simulink model "SimulationSorting"  (R2024b)
settings: Solver=VariableStepAuto  StartTime=0.0  StopTime=Inf  RelTol=1e-3
PreLoadFcn:
  | addpath(genpath(pwd))
  | load("model_data.mat");
undefined symbols (not defined in the file): gray, q_grip1, Sim3dSensor
libraries: sim3dlib x5, robotcorelib x1, robotmaniplib x1, sim3dcameralib x1, robotsim3dlib x1
settings Model: Creator=gbhosale  LastModifiedBy=10177

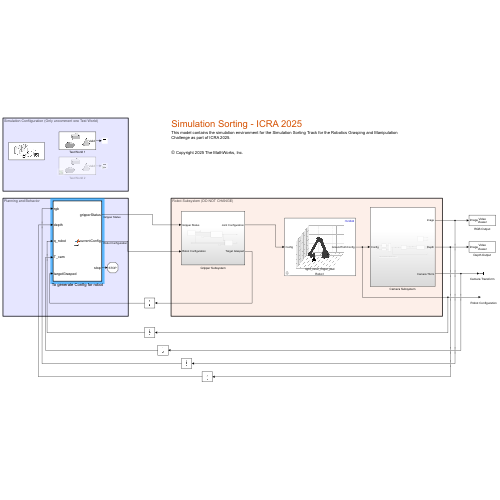
[thumbnail: Simulink's stored preview of the top-level diagram]
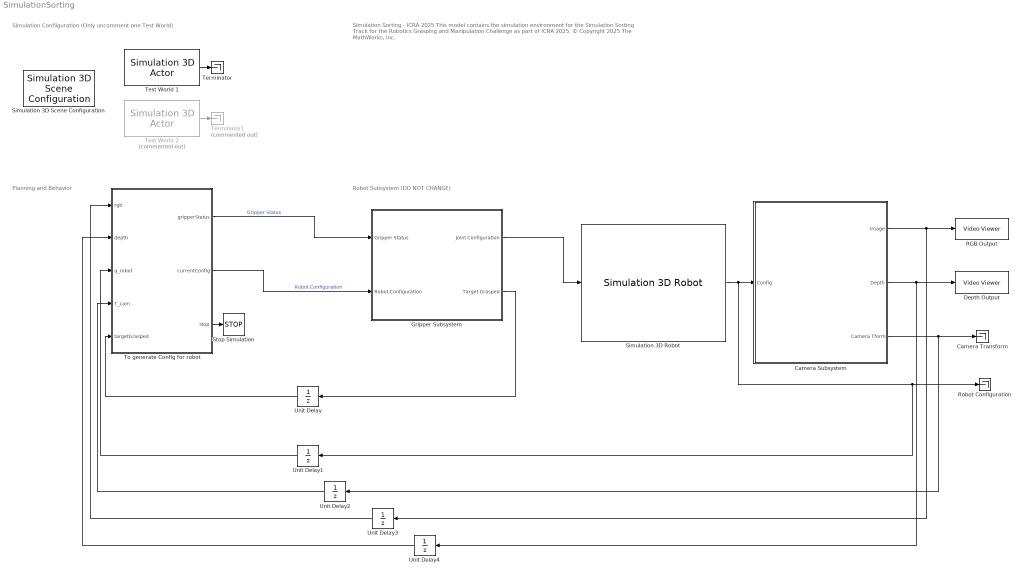
== system SimulationSorting ==
  note: Robot Subsystem (DO NOT CHANGE)
  note: Planning and Behavior
  note: Simulation Confiiguration (Only uncomment one Test World)
  note: Simulation Sorting - ICRA 2025
      | This model contains the simulation environment for the Simulation Sorting Track for the Robotics Grasping and Manipulation Challenge as part of ICRA 2025.
      |
      | © Copyright 2025 The MathWorks, Inc.
  Camera Subsystem : Subsystem
  Camera Transform : Terminator
  Depth Output : VideoViewer  colormapValue=gray(256)  FigPos=[886.5 747 400.5 311]
  Gripper Subsystem : Subsystem
  RGB Output : VideoViewer  colormapValue=gray(256)  FigPos=[892.5 410 400 305]
  Robot Configuration : Terminator
  Simulation 3D Robot : robotsim3dlib/Simulation 3D Robot  actorInputType=RigidBodyTree Object  RigidBodyTree=rt.robot  ActorName=Robo1  existActorChekBox=on  initialTrans=[nan nan nan]  initialRot=[ 0 0 0]  initialConfig=[-0.2618 -2.1991 1.9722 -1.3963 -1.5882 1.3265 0 0 0 0 0 0]  EndEffector=right_inner_finger_pad  eeOffsetInpChekBox=off  eeTargetTrans=[ 0 0 0.08 ]  eeTargetRot=[ 0 0 0 ]  enableRegionGraspChekBox=off  regionGraspInpChekBox=on  eeTargTransDiff=[ 0.001 0.001 2 ]  eeTargRotDiff=[ nan nan nan ]  inpConfEnbVal=on  inpGraspEnbVal=off  inpTransEnbVal=off  outConfEnbVal=on  outGraspEnbVal=off  outTransEnbVal=off  SampleTime=0.01  ActorType=SimulinkVehicle  ID=C  aMode=6  ActorTag=Robo1  Mesh=RigidBodyTree
  Simulation 3D Scene Configuration : sim3dlib/Simulation 3D Scene Configuration  Priority=0  ProjectFormat=Unreal Executable  SceneDesc=Empty scene  ProjectName=SimSort_Env_Executable\VehicleSimulation.exe  ScenePath=/Game/Maps/EmptyScene  EnableOpenDRIVE=off  vehTagList={'Custom';'Robo1';'Scene Origin';'Sim3dActor2';'Sim3dActor3';'SimSortWorld';'cameraPlaceHolder'}  vehTag=Scene Origin  FreeCameraInitialTranslation=[0, 0, 0]  FreeCameraDefaultInitialTranslation=[-6, 0, 2]  FreeCameraInitialRotation=[0, 0, 0]  FreeCameraDefaultInitialRotation=[0, -15, 0]  OpVisEn=off  Ts=0.01  EnableWindow=on  EnableRemoteAccess=off  EnableWeather=off  SunAzimuth=90  SunAltitude=40.0  EnableGeospatialSun=off  Latitude=0  Longitude=0  Date=2023-01-01  Time=10:30:00  GeoTimeZone=-5.0  SunDaylightSaving=off  wind=1  clouds=10  EnableVolumetricClouds=off  CloudCoverage=0  CloudAltitude=6  fog=0  rain=0  RaindropsEffect=off  SnowDensity=0  EnableGeospatial=off  UseTrueOrigin=off  OriginHeight=200  OriginLatitude=40.744652  OriginLongitude=-73.988864  MapStyle=Aerial  AdditionalAssetIDs=[]  UseAdvancedSunSky=off  SolarTime=11  TimeZone=-5  Day=21  Month=9  Year=2022  UseDaylightSavingTime=on  DSTStartDay=10  DSTStartMonth=3  DSTEndDay=3  DSTEndMonth=11  DSTSwitchHour=2  sensorTag=MainCamera1  sensorId=1  sensorName=MainCamera1  mountLoc=Origin  offsetFlag=off  tmountOffset=[0, 0, 0]  rmountOffset=[0, 0, 0]  HorizontalResolution=1280  VerticalResolution=720  HorizontalFOV=60  mountPoint=[0 0 0]  mountOrientation=[0 0 0]  aMode=6  ID=1  GeoTrigger=Inactive
      settings: LibrarySourceBlock=robotsim3dlib/Simulation 3D Scene Configuration
  Stop Simulation : Stop
  Terminator : Terminator
  Terminator1 : Terminator  Commented=on
  Test World 1 : sim3dlib/Simulation 3D Actor  Priority=1  ActorName=SimSortWorld  ParentName=Scene Origin  Operation=Create at setup  InitScriptText=|  SampleTime=-1  Translation=[0 0 0]  Rotation=[0 0 0]  Scale=[1 1 1]  aMode=5  ActorTag=SimSortWorld  ActorType=Sim3dActor  ID=C
      | % Reserved keywords:
      | % - Actor : handle to this actor object
      | % - World : handle to the world object
      | 
      | % Examples:
      | 
      | % Create a primitive geometry (optional)
      | % createShape(Actor, 'box', [1 1 1]);
      | 
      | % Initialize values (optional)
      | % Actor.Physics = true;
      | % Actor.Color = [1 0 0];
      | 
      | Actor.load('simSortWorld1.mat')
  Test World 2 : sim3dlib/Simulation 3D Actor  Priority=1  Commented=on  ActorName=Sim3dActor3  ParentName=Scene Origin  Operation=Create at setup  InitScriptText=|  SampleTime=-1  Translation=[0 0 0]  Rotation=[0 0 0]  Scale=[1 1 1]  aMode=5  ActorTag=Sim3dActor3  ActorType=Sim3dActor  ID=3
      | % Reserved keywords:
      | % - Actor : handle to this actor object
      | % - World : handle to the world object
      | 
      | % Examples:
      | 
      | % Create a primitive geometry (optional)
      | % createShape(Actor, 'box', [1 1 1]);
      | 
      | % Initialize values (optional)
      | % Actor.Physics = true;
      | % Actor.Color = [1 0 0];
      | 
      | Actor.load('simSortWorld2.mat')
  To generate Config for robot : MATLAB Function  TreatAsAtomicUnit=on
  Unit Delay{,1..4} (5 alike) : UnitDelay  SampleTime=-1  HasFrameUpgradeWarning=on
  wires:
  To generate Config for robot/3(stop) -> Stop Simulation/1
  Simulation 3D Robot/1 -> Camera Subsystem/1(Config), Unit Delay1/1, Robot Configuration/1
  Test World 1/1 -> Terminator/1
  Test World 2/1 -> Terminator1/1
  To generate Config for robot/1(gripperStatus) -> Gripper Subsystem/1(Gripper Status)  "Gripper Status"
  To generate Config for robot/2(currentConfig) -> Gripper Subsystem/2(Robot Configuration)  "Robot Configuration"
  Gripper Subsystem/1(Joint Configuration) -> Simulation 3D Robot/1
  Gripper Subsystem/2(Target Grasped) -> Unit Delay/1
  Unit Delay/1 -> To generate Config for robot/5(targetGrasped)
  Camera Subsystem/1(Image) -> Unit Delay3/1, RGB Output/1
  Camera Subsystem/2(Depth) -> Unit Delay4/1, Depth Output/1
  Camera Subsystem/3(Camera Tform) -> Unit Delay2/1, Camera Transform/1
  Unit Delay1/1 -> To generate Config for robot/3(q_robot)
  Unit Delay2/1 -> To generate Config for robot/4(T_cam)
  Unit Delay4/1 -> To generate Config for robot/2(depth)
  Unit Delay3/1 -> To generate Config for robot/1(rgb)

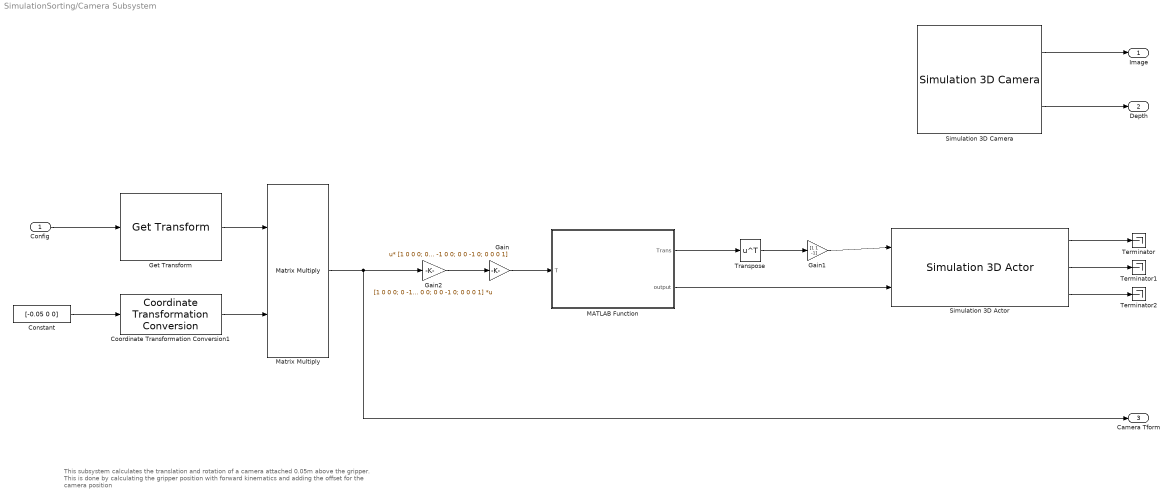
== system SimulationSorting/Camera Subsystem ==
  note: This subsystem calculates the translation and rotation of a camera attached 0.05m above the gripper. This is done by calculating the gripper position with forward kinematics and adding the offset for the camera position
  Config : Inport
  Constant : Constant  Value=[-0.05 0 0]
  Coordinate Transformation Conversion1 : robotcorelib/Coordinate Transformation Conversion  InputRepresentation=Translation Vector  InputEulerSequence=ZYX  ShowTrVecInputPort=on  OutputRepresentation=Homogeneous Transformation  OutputEulerSequence=ZYX  ShowTrVecOutputPort=on  SimulateUsing=Interpreted execution
  Gain : Gain  Gain=[1 0 0 0; 0 -1 0 0; 0 0 -1 0; 0 0 0 1]  Multiplication=Matrix(u*K)
  Gain1 : Gain  Gain=[1 1 -1]
  Gain2 : Gain  Gain=[1 0 0 0; 0 -1 0 0; 0 0 -1 0; 0 0 0 1]  Multiplication=Matrix(K*u)
  Get Transform : robotmaniplib/Get Transform  RigidBodyTree=rt.robot  SourceBody=robotiq_arg2f_base_link  TargetBody=base_link  SimulateUsing=Interpreted execution
  MATLAB Function : MATLAB Function  TreatAsAtomicUnit=on
  Matrix Multiply : Product  Multiplication=Matrix(*)
  Simulation 3D Actor : sim3dlib/Simulation 3D Actor  Priority=1  ActorName=cameraPlaceHolder  ParentName=Robo1  Operation=Create at setup  InitScriptText=|  SampleTime=-1  Translation=[0.05 0 0]  Rotation=[0 0 0]  Scale=[1 1 1]  InputsText=cameraPlaceHolder.Translation cameraPlaceHolder.Rotation  OutputsText=cameraPlaceHolder.Translation cameraPlaceHolder.Rotation  aMode=5  ActorTag=cameraPlaceHolder  ActorType=Sim3dActor  ID=C
      | Actor.createShape('box', [0.02 0.04 0.06]);
      | Actor.Mobility=sim3d.utils.MobilityTypes.Movable;
      | Actor.Color=[1 0 0];
      | Actor.Translation=[0.05, 0, 0];
      | Actor.Rotation = [0, 0, 0];
      | Actor.ConstantAttributes=false;
      | Actor.Mass = 1;
      | Actor.Transparency = 0;
      | Actor.Shininess = 0;
  Simulation 3D Camera : sim3dcameralib/Simulation 3D Camera  Priority=1  sensorTag=Sim3dSensor�  sensorId=3  sensorName=Sim3dSensor�  vehTagList={'Robo1';'Scene Origin';'Sim3dActor2';'Sim3dActor3';'SimSortWorld';'cameraPlaceHolder'}  vehTag=cameraPlaceHolder  mountLoc=Origin  offsetFlag=on  tmountOffset=[0 0 0]  extTmount=off  rmountOffset=[0, -90, 0]  extRmount=off  FocalLength=[1109, 1109]  OpticalCenter=[640, 360]  ImageSize=[720, 1280]  RadialDistortion=[0, 0]  TangentialDistortion=[0, 0]  SensorSkew=0  DepthOutportEnabled=on  SemanticOutportEnabled=off  TransformOutportEnabled=off  SampleTime=0.01  mountPoint=[0 0 0]  mountOrientation=[0 90 0]  aMode=5  ID=3
      settings: LibrarySourceBlock=Simulation 3D Camera
  Terminator : Terminator
  Terminator1 : Terminator
  Terminator2 : Terminator
  Transpose : Math  Operator=transpose
  Image : Outport
  Depth : Outport  Port=2
  Camera Tform : Outport  Port=3
  wires:
  Config/1 -> Get Transform/1
  Coordinate Transformation Conversion1/1 -> Matrix Multiply/2
  Get Transform/1 -> Matrix Multiply/1
  Constant/1 -> Coordinate Transformation Conversion1/1
  Matrix Multiply/1 -> Camera Tform/1, Gain2/1
  Simulation 3D Camera/1 -> Image/1
  Simulation 3D Camera/2 -> Depth/1
  Gain2/1 -> Gain/1
  Gain/1 -> MATLAB Function/1(T)
  MATLAB Function/1(Trans) -> Transpose/1
  Transpose/1 -> Gain1/1
  Gain1/1 -> Simulation 3D Actor/1
  MATLAB Function/2(output) -> Simulation 3D Actor/2
  Simulation 3D Actor/3 -> Terminator2/1
  Simulation 3D Actor/2 -> Terminator1/1
  Simulation 3D Actor/1 -> Terminator/1

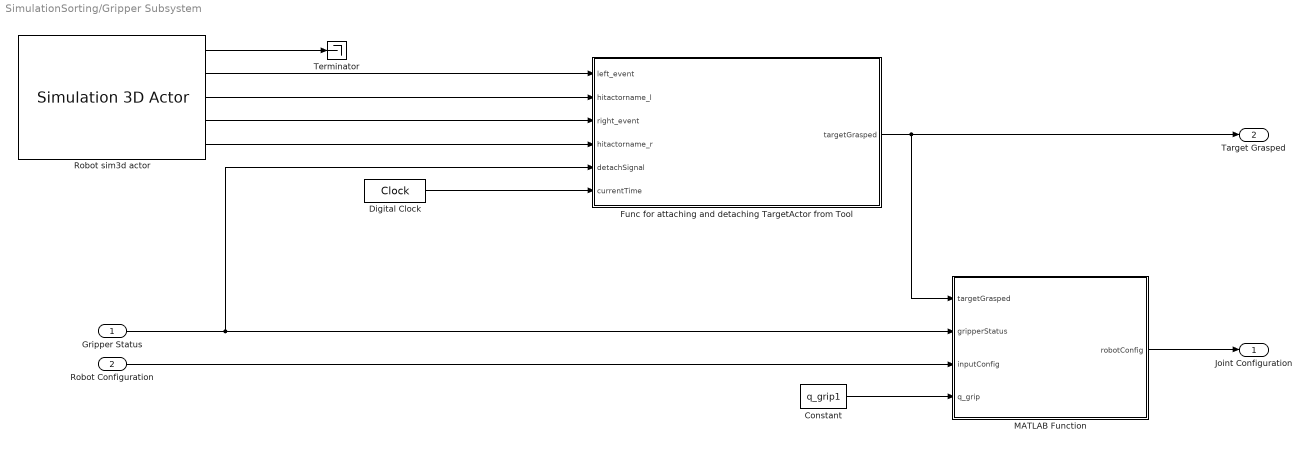
== system SimulationSorting/Gripper Subsystem ==
  Gripper Status : Inport
  Robot Configuration : Inport  Port=2
  Constant : Constant  Value=q_grip1
  Digital Clock : DigitalClock  SampleTime=0.01
  Func for attaching and detaching TargetActor from Tool : MATLAB Function  TreatAsAtomicUnit=on
  MATLAB Function : MATLAB Function  TreatAsAtomicUnit=on
  Robot sim3d actor : sim3dlib/Simulation 3D Actor  Priority=1  ActorName=Sim3dActor2  ParentName=Scene Origin  Operation=Create at setup  InitScriptText=|  SampleTime=-1  Translation=[0 0 0]  Rotation=[0 0 0]  Scale=[1 1 1]  EventsText=|  aMode=5  ActorTag=Sim3dActor2  ActorType=Sim3dActor  ID=2
      InitScriptText=|
      | rt = load('ur5e_gripper.mat');
      | robotActor = sim3d.Actor('ActorName', 'Robo1');
      | World.add(robotActor,Actor);
      | 
      | robotActor.load(rt.robot,[1 1 1]);
      | 
      | % finding tool reference 
      | tool1 = World.Actors.left_inner_finger_pad;
      | tool2 = World.Actors.right_inner_finger_pad;
      | tool1.HitEventEnabled = true;
      | tool1.Collisions = true;
      | 
      | tool2.HitEventEnabled = true;
      | tool2.Collisions = true;
      | 
      | %tool1.Physics = true; % somehow this Phsyics dont work
      | % tool1.Color = [10 0 0];
      | tool1.Mobility =  sim3d.utils.MobilityTypes.Movable;
      | 
      | % tool2.Color = [10 0 0];
      | tool2.Mobility =  sim3d.utils.MobilityTypes.Movable;
      | 
      | propagate(World.Actors.('Sim3dActor2'),'Mobility', sim3d.utils.MobilityTypes.Movable);
      | propagate(World.Actors.('Sim3dActor2'),'Shadows',true);
      EventsText=|
      | left_inner_finger_pad.HitEvent          
      | left_inner_finger_pad.HitOtherActorName 
      | right_inner_finger_pad.HitEvent         
      | right_inner_finger_pad.HitOtherActorName
  Terminator : Terminator
  Joint Configuration : Outport
  Target Grasped : Outport  Port=2
  wires:
  Func for attaching and detaching TargetActor from Tool/1(targetGrasped) -> Target Grasped/1, MATLAB Function/1(targetGrasped)
  Digital Clock/1 -> Func for attaching and detaching TargetActor from Tool/6(currentTime)
  Gripper Status/1 -> Func for attaching and detaching TargetActor from Tool/5(detachSignal), MATLAB Function/2(gripperStatus)
  Robot sim3d actor/2 -> Func for attaching and detaching TargetActor from Tool/1(left_event)
  Robot sim3d actor/3 -> Func for attaching and detaching TargetActor from Tool/2(hitactorname_l)
  Robot sim3d actor/4 -> Func for attaching and detaching TargetActor from Tool/3(right_event)
  Robot sim3d actor/5 -> Func for attaching and detaching TargetActor from Tool/4(hitactorname_r)
  Robot Configuration/1 -> MATLAB Function/3(inputConfig)
  Constant/1 -> MATLAB Function/4(q_grip)
  MATLAB Function/1(robotConfig) -> Joint Configuration/1
  Robot sim3d actor/1 -> Terminator/1

== matlab function SimulationSorting/Gripper Subsystem/Func for attaching and detaching TargetActor from Tool ==
  data: left_event input; hitactorname_l input; right_event input; hitactorname_r input; detachSignal input double; targetGrasped output; currentTime input
 function targetGrasped = fcn(left_event, hitactorname_l, right_event, hitactorname_r, detachSignal, currentTime)
    
    persistent l_time r_time grasped;
    if isempty(l_time)
        l_time = 0;
    end

    if isempty(r_time)
        r_time = 1;
    end

    if left_event
        l_time = currentTime;
    end

    if right_event
        r_time = currentTime;
    end
    
    if isempty(grasped)
        grasped = 0;
    end

    targetGrasped = grasped;

    coder.extrinsic('attachToTool');

    if abs(l_time - r_time) < 0.5 || ~detachSignal
        grasped = attachToTool(hitactorname_l, hitactorname_r,detachSignal);
        targetGrasped = grasped;
    end
end

== matlab function SimulationSorting/To generate Config for robot ==
  data: rgb input; depth input; q_robot input; T_cam input; gripperStatus output; currentConfig output size=[6 1]; stop output; targetGrasped input
function [gripperStatus, currentConfig, stop]  = main(rgb, depth, q_robot, T_cam, targetGrasped)

coder.extrinsic('imwrite');
stop = false;
gripperStatus = 0; % 0 = Open; 1 = Close
get_photo_poses = [0.025 -0.752 0.57 pi 0 pi/2;
                   0.35 -0.2 0.7 pi 0 pi/2;   
                   0.1 -0.2 0.7 pi 0 pi/2;    
                   -0.35 -0.25 0.7 pi 0 pi/2;   
                   % 0.4 -0.63 0.65 pi 0 pi/2;
                   0.4 -0.63 0.575 pi 0 pi/2
                   0.0 -0.63 0.68 pi 0 pi/2;
                   -0.3 -0.63 0.63 pi 0 pi/2;]; % out of range, static area, orientation, bin-picking, objects change one/two/three
valid_range = [-0.4, 0.4, -0.3, -0.1;
               -0.4, 0.01, -0.3, 0.3;
               -0.24, 0.32, -0.3, 0.15;
               -0.085, 0.085, -0.127, 0.127;
               -0.4, 0.4, -0.3, 0.3;
               -0.4, 0.4, -0.3, 0.3;
               -0.4, 0.4, -0.3, 0.3;]; % [x_min x_max y_min y_max] valid range for photo
place_poses = [-0.32 0.5 0.45 pi 0 -pi/2;
               0.0 0.5 0.45 pi 0 -pi/2; 
               0.32 0.5 0.45 pi 0 -pi/2]; % r g b region
out_range_poses = [0.185, -0.8404, 0.1576, pi, pi/4, pi/2;
                   0.235, -0.8404, 0.1576, pi, pi/4, pi/2;
                   0.285, -0.8404, 0.1576, pi, pi/4, pi/2;];
approach_z = 0.1;

persistent index delay cur_q traj is_planned grasp_pose tar_area photo_id place_pose out_range_id out_range_classes numObjects;
if isempty(index)
    index = 1;
end

if isempty(out_range_id)
    out_range_id = 1;
end

if isempty(numObjects)
    numObjects = 0;
end

if isempty(out_range_classes)
    out_range_classes = zeros(1, 3);
end

if isempty(photo_id)
    photo_id = 1;
end

if isempty(tar_area) 
    tar_area = 1;
end

if isempty(delay)
    delay = 1;
end

if isempty(cur_q)
    cur_q = [-0.8562 -1.6827 1.1032 -0.9913 -1.5708 2.2854];
end

if isempty(is_planned)
    is_planned = false;
end

if isempty(traj)
    traj = zeros(6, 1);
end

if isempty(grasp_pose)
    grasp_pose = [-0.2099 -0.5817 0.2291 pi 0 pi];
end

if isempty(place_pose)
    place_pose = place_poses(1, :);
end

% States to pick and place. 1 = INIT; 2 = GO_HOME; 2 = CHOOSE_OBJECT; 3 = REACH; 4 = APPROACH; 5 = GRAB; 6 = LIFT; 7 = PLACE; 8 = DROP; 9 = GO_HOME 
% 10 = End Simulation

persistent state;
if isempty(state)
    state = 1;
end

persistent ik weights chomp ur5e initialguess;
if isempty(chomp)
    ur5e = importrobot("universalUR5e.urdf", 'DataFormat', 'row', 'MaxNumBodies',24);

    shoulder_link = getBody(ur5e, "shoulder_link");
    newJoint = copy(shoulder_link.Joint);
    newJoint.PositionLimits = [-pi, pi];
    replaceJoint(ur5e, "shoulder_link", newJoint);

    upper_arm_link = getBody(ur5e, "upper_arm_link");
    newJoint = copy(upper_arm_link.Joint);
    newJoint.PositionLimits = [-pi, 0];
    replaceJoint(ur5e, "upper_arm_link", newJoint); % [-pi, 0]

    forearm_link = getBody(ur5e, 'forearm_link');
    newJoint = copy(forearm_link.Joint);
    newJoint.PositionLimits = [0, pi];
    replaceJoint(ur5e, "forearm_link", newJoint); % [0, pi]

    wrist_1_link = getBody(ur5e, 'wrist_1_link');
    newJoint = copy(wrist_1_link.Joint);
    newJoint.PositionLimits = [-pi, 0];
    replaceJoint(ur5e, "wrist_1_link", newJoint); % [-pi, 0]

    wrist_2_link = getBody(ur5e, 'wrist_2_link');
    newJoint = copy(wrist_2_link.Joint);
    newJoint.PositionLimits = [-pi, 0];
    replaceJoint(ur5e, "wrist_2_link", newJoint); % [-pi, 0]

    wrist_3_link = getBody(ur5e, 'wrist_3_link');
    newJoint = copy(wrist_3_link.Joint);
    newJoint.PositionLimits = [-pi, pi];
    replaceJoint(ur5e, "wrist_3_link", newJoint); % [-pi, pi]

    initialguess = [-1.87 -1.31 1.82 -2.10 -1.57 0.88];
    ik = inverseKinematics("RigidBodyTree", ur5e);
    ik.SolverParameters.EnforceJointLimits = true;
    weights = [0.25, 0.25, 0.25, 1, 1, 1];
    chomp = manipulatorCHOMP(ur5e);
    % chomp.CollisionOptions.IgnoreSelfCollision = false;
end

if state ~= 1
    cur_q = q_robot(1, 1:6);
    cur_T = getTransform(ur5e, cur_q, 'tool0');
    cur_ee = hom2euler(cur_T);
    cur_cam = hom2euler(T_cam);
    disp("cur_q:");
    disp(cur_q);
    disp("state:");
    disp(state);
    disp("cur_ee:");
    disp(cur_ee);
    disp("cur_cam:");
    disp(cur_cam);
end

if state == 1 % INIT
    index = index + 1;
    gripperStatus = 0;
    currentConfig = cur_q';
    if index > 10
        index = 1;
        state = 2;
    end
elseif state == 2 % GO_HOME
    if is_planned == false
        traj = PathPlanning(chomp, ik, weights, initialguess, cur_q, get_photo_poses(tar_area, :))';
        is_planned = true;
    end
    gripperStatus = 0;
    currentConfig = traj(1:6, index);
    index = index + 1;
    if index > size(traj, 2)
        is_planned = false;
        state = 3;
        index = 1;
    end
elseif state == 3 % CHOOSE_OBJECT
    rgb_filename = sprintf('Logs\\rgb%d.png', int32(photo_id));
    depth_filename = sprintf('Logs\\depth%d.png', int32(photo_id));
    depth_data_filename = sprintf('Logs\\depth_data%d.mat', int32(photo_id));
    imwrite(rgb, rgb_filename);
    imwrite(depth, depth_filename);
    save(depth_data_filename, 'depth', '-v7.3');
    
    %%% calc grasp pose by rgb and depth
    class = 0;
    if tar_area == 1
        if out_range_id == 1
            [out_range_classes, numObjects] = OutRangeDetect(depth, rgb, valid_range(tar_area, :));
        else
            numObjects = numObjects - 1;
        end

        if numObjects > 0
            grasp_pose = out_range_poses(out_range_id, :);
            class = out_range_classes(out_range_id);
            out_range_id = out_range_id + 1;
        end
    else
        cur_cam = hom2euler(T_cam);
        [grasp_pose, class, numObjects] = GraspPlanning(depth, rgb, cur_cam, valid_range(tar_area, :), 1, photo_id);
    end
    disp("num_objects:");
    disp(numObjects);

    is_planned = false;
    photo_id = photo_id + 1;
    gripperStatus = 0;
    currentConfig = cur_q';
    if numObjects == 0
        if tar_area == 7
            state = 10; % stop
        else
            tar_area = mod(tar_area, 7) + 1;
            state = 2;
        end
    else
        if class == 4 || class == 5 || class == 6
            place_pose = place_poses(1, :);
        elseif class == 3 || class == 7
            place_pose = place_poses(2, :);
        else
            place_pose = place_poses(3, :);
        end
        state = 4;
    end
elseif state == 4 % REACH
    if is_planned == false
        if tar_area == 1
            reach_pose = grasp_pose + [0 approach_z approach_z 0 0 0];
        else
            reach_pose = grasp_pose + [0 0 approach_z 0 0 0];
        end
        traj = PathPlanning(chomp, ik, weights, initialguess, cur_q, reach_pose)';
        is_planned = true;
    end
    gripperStatus = 0;
    currentConfig = traj(1:6, index);
    index = index + 1;
    if index > size(traj, 2)
        is_planned = false;
        state = 5;
        index = 1;
    end
elseif state == 5 % APPROACH
    if is_planned == false
        traj = PathPlanning(chomp, ik, weights, initialguess, cur_q, grasp_pose)';
        is_planned = true;
    end
    gripperStatus = 0;
    currentConfig = traj(1:6, index);
    index = index + 1;
    if index > size(traj, 2)
        is_planned = false;
        state = 6;
        index = 1;
    end    
elseif state == 6 % GRAB
    gripperStatus = 1;
    currentConfig = cur_q';
    index = index + 1;
    if index > 60
        state = 7;
        index = 1;
    end
    if targetGrasped
        state = 7;
        index = 1;
    end
elseif state == 7 % LIFT
    if is_planned == false
        if tar_area == 1
            lift_pose = grasp_pose + [0 2*approach_z 3*approach_z 0 0 0];
        else
            lift_pose = grasp_pose + [0 0 approach_z 0 0 0];
        end
        traj = PathPlanning(chomp, ik, weights, initialguess, cur_q, lift_pose)';
        is_planned = true;
    end
    gripperStatus = 1;
    currentConfig = traj(1:6, index);
    index = index + 1;
    if index > size(traj, 2)
        is_planned = false;
        state = 8;
        index = 1;
    end
elseif state == 8 % PLACE
    if is_planned == false
        traj = PathPlanning(chomp, ik, weights, initialguess, cur_q, place_pose)';
        is_planned = true;
    end
    gripperStatus = 1;
    currentConfig = traj(1:6, index);
    index = index + 1;
    if index > size(traj, 2)
        is_planned = false;
        state = 9;
        index = 1;
    end
elseif state == 9 % DROP
    gripperStatus = 0;
    currentConfig = cur_q';
    index = index + 1;
    if index > 60
        state = 2;
        index = 1;
    end
else
    currentConfig = cur_q';
    stop = true;
end

end

function traj = PathPlanning(chomp, ik, weights, initialguess, cur_q, target_pose)

    translation = target_pose(1:3);
    eulerAngles = [target_pose(6) target_pose(5) target_pose(4)];

    T = eul2tform(eulerAngles,"ZYX");
    T(1:3, 4) = translation;

    [tar_q, ~] = ik('tool0', T, weights, initialguess);
    timepoints = [0 1];
    timestep = 0.02;
    trajtype = "minjerkpolytraj";
    [traj, ~] = optimize(chomp, [cur_q; tar_q], timepoints, timestep, InitialTrajectoryFitType=trajtype);

    disp("tar_q:");
    disp(tar_q);
    disp("tar_pose:");
    disp(target_pose);
end

function [grasp_pose, class, numObjects] = GraspPlanning(depth, rgb, cur_cam, cropped_range, prior_id, photo_id)
    minPoints = 50;
    depth_data = depth;
    fx = 1109.0;
    fy = 1109.0;
    cx = 640.0;
    cy = 360.0;
    
    % register pointcloud 
    validIdx = depth_data > 0.2 & depth_data < 0.9;
    [rows, cols] = size(depth_data);
    [u, v] = meshgrid(1:cols, 1:rows);
    X = (u - cx) .* depth_data / fx;
    Y = (v - cy) .* depth_data / fy;
    Z = depth_data;
    points3D = [X(validIdx), Y(validIdx), Z(validIdx)];
    colors = reshape(rgb, [], 3); 
    colors = colors(validIdx, :); 
    ptCloud = pointCloud(points3D, 'Color', colors);

    % extract ground
    [~, inliers] = pcfitplane(ptCloud, 0.001);
    groundCloud = select(ptCloud, inliers);
    outliers = setdiff(1:ptCloud.Count, inliers);
    foreCloud = select(ptCloud, outliers);

    % filter invalid area
    validPoints = foreCloud.Location(:,1) >= cropped_range(1) & ...
                  foreCloud.Location(:,1) <= cropped_range(2) & ...
                  foreCloud.Location(:,2) >= cropped_range(3) & ...
                  foreCloud.Location(:,2) <= cropped_range(4);
    validCloud = select(foreCloud, validPoints);

    % cluster
    [labels, numClusters] = pcsegdist(validCloud, 0.01);
    clusterClouds = cell(1, numClusters);
    for i = 1:numClusters
        clusterIndices = (labels == i);
        clusterClouds{i} = validCloud.Location(clusterIndices, :);
    end

    clusterCenters = zeros(numClusters, 2);
    clusterZ = zeros(numClusters, 1);
    pointCounts = zeros(numClusters, 1);
    for i = 1:numClusters
        clusterPoints = clusterClouds{i};
        clusterCenters(i, :) = mean(clusterPoints(:,1:2), 1);
        clusterZ(i, :) = mean(clusterPoints(:, 3), 1);
        size_pc = size(clusterPoints);
        pointCounts(i) = size_pc(1);
    end

    % filter min points noisy
    validClusters = (pointCounts >= minPoints);
    objectClouds = cell(1, 0);
    for i = 1:numClusters
        if validClusters(i)
            objectClouds{end + 1} = clusterClouds{i};
        end
    end
    objectCenters = clusterCenters(validClusters, :);
    objectZ = clusterZ(validClusters, :);
    numObjects = numel(objectClouds);
    if numObjects == 0
        grasp_pose = zeros(1, 6);
        class = 0;
        return;
    end

    %%% select target object and calc its feature

    % % distance to img center
    % norms = vecnorm(objectCenters, 2, 2);
    % [~, sortIdx] = sort(norms);
    % selectedIdx = sortIdx(prior_id);
    % targetCloudLocation = objectClouds{selectedIdx};
    % targetCloud = pointCloud(targetCloudLocation);

    % distance to camera
    [~, sortIdx] = sort(objectZ);
    selectedIdx = sortIdx(prior_id);
    targetCloudLocation = objectClouds{selectedIdx};
    targetCloud = pointCloud(targetCloudLocation);    

    % extract plane
    [~, inliers] = pcfitplane(targetCloud, 0.005, [0 0 1]);
    planeCloud = select(targetCloud, inliers);

    % calc pca
    [coeff, ~] = pca(planeCloud.Location);
    second_axis = coeff(:,2)'; 
    center = mean(planeCloud.Location, 1);

    %%% classification

    % get object image
    points3D = targetCloudLocation;  
    u = (points3D(:,1) .* fx) ./ points3D(:,3) + cx;
    v = (points3D(:,2) .* fy) ./ points3D(:,3) + cy;
    uv = round([u, v]);
    
    validIndices = uv(:,1) >= 1 & uv(:,1) <= size(rgb,2) & ...
                   uv(:,2) >= 1 & uv(:,2) <= size(rgb,1);
    uvValid = uv(validIndices, :);

    mask = false(size(rgb,1), size(rgb,2));
    linearIndices = sub2ind(size(mask), uvValid(:,2), uvValid(:,1));
    mask(linearIndices) = true;

    xMin = max(min(uvValid(:,1)), 1);
    xMax = min(max(uvValid(:,1)), size(rgb,2));
    yMin = max(min(uvValid(:,2)), 1);
    yMax = min(max(uvValid(:,2)), size(rgb,1));
    bboxWidth = xMax - xMin + 1;
    bboxHeight = yMax - yMin + 1;

    maskedImg = rgb;
    bgColor = [11, 20, 43];
    for c = 1:3
        channel = maskedImg(:,:,c);
        channel(~mask) = bgColor(c);
        maskedImg(:,:,c) = channel;
    end
    
    cropped = imcrop(maskedImg, [xMin, yMin, bboxWidth-1, bboxHeight-1]);
    
    squareSize = max(bboxWidth, bboxHeight);
    squareImg = repmat(reshape(uint8(bgColor),1,1,3), squareSize, squareSize, 1);
    
    xOffset = floor((squareSize - bboxWidth)/2);
    yOffset = floor((squareSize - bboxHeight)/2);
    
    squareImg(yOffset+1:yOffset+bboxHeight,...
             xOffset+1:xOffset+bboxWidth, :) = cropped;
    
    resized_size = [227 227];
    resizedImg = imresize(squareImg, resized_size, 'bilinear');  
    
    % run cnn
    class = classifier(resizedImg);

    coder.extrinsic('imwrite');
    rgb_filename = sprintf('Logs\\object%d_%d.png', int32(photo_id), int32(class));
    imwrite(resizedImg, rgb_filename);

    %%% calc grasp pose
    v_proj = [second_axis(1), second_axis(2), 0];
    theta = atan2(-v_proj(1), -v_proj(2));
    if theta > pi/2 % [-pi/2, pi/2]
        theta = theta - pi;
    elseif theta < -pi/2
        theta = theta + pi;
    end    

    % grasp depth adjustment
    target_z = cur_cam(3) - center(3);
    if class == 6
        tool_gripper_dist = 0.145;
    elseif target_z > 0.07
        tool_gripper_dist = 0.125;
    else
        tool_gripper_dist = 0.14;
    end

    grasp_pose = [cur_cam(1) - center(1), ...
                  cur_cam(2) + center(2), ...
                  target_z + tool_gripper_dist, ...
                  cur_cam(4), ...
                  cur_cam(5), ...
                  theta];

    disp("grasp_pose:");
    disp(grasp_pose);
end

function [out_range_classes, numObjects] = OutRangeDetect(depth, rgb, cropped_range)
    coder.extrinsic('imwrite');
    minPoints = 50;
    depth_data = depth;
    fx = 1109.0;
    fy = 1109.0;
    cx = 640.0;
    cy = 360.0;
    
    % register pointcloud 
    validIdx = depth_data > 0.2 & depth_data < 0.9;
    [rows, cols] = size(depth_data);
    [u, v] = meshgrid(1:cols, 1:rows);
    X = (u - cx) .* depth_data / fx;
    Y = (v - cy) .* depth_data / fy;
    Z = depth_data;
    points3D = [X(validIdx), Y(validIdx), Z(validIdx)];
    colors = reshape(rgb, [], 3); 
    colors = colors(validIdx, :); 
    ptCloud = pointCloud(points3D, 'Color', colors);

    % extract ground
    [~, inliers] = pcfitplane(ptCloud, 0.001);
    groundCloud = select(ptCloud, inliers);
    outliers = setdiff(1:ptCloud.Count, inliers);
    foreCloud = select(ptCloud, outliers);

    % filter invalid area
    validPoints = foreCloud.Location(:,1) >= cropped_range(1) & ...
                  foreCloud.Location(:,1) <= cropped_range(2) & ...
                  foreCloud.Location(:,2) >= cropped_range(3) & ...
                  foreCloud.Location(:,2) <= cropped_range(4);
    validCloud = select(foreCloud, validPoints);

    % cluster
    [labels, numClusters] = pcsegdist(validCloud, 0.01);
    clusterClouds = cell(1, numClusters);
    for i = 1:numClusters
        clusterIndices = (labels == i);
        clusterClouds{i} = validCloud.Location(clusterIndices, :);
    end

    clusterCenters = zeros(numClusters, 2);
    clusterZ = zeros(numClusters, 1);
    pointCounts = zeros(numClusters, 1);
    for i = 1:numClusters
        clusterPoints = clusterClouds{i};
        clusterCenters(i, :) = mean(clusterPoints(:,1:2), 1);
        clusterZ(i, :) = mean(clusterPoints(:, 3), 1);
        size_pc = size(clusterPoints);
        pointCounts(i) = size_pc(1);
    end

    % filter min points noisy
    validClusters = (pointCounts >= minPoints);
    objectClouds = cell(1, 0);
    for i = 1:numClusters
        if validClusters(i)
            objectClouds{end + 1} = clusterClouds{i};
        end
    end
    objectCenters = clusterCenters(validClusters, :);
    numObjects = numel(objectClouds);
    if numObjects == 0
        out_range_classes = zeros(1, 3);
        return;
    end

    % distance to img center
    norms = vecnorm(objectCenters, 2, 2);
    [~, sortIdx] = sort(norms);

    %%% classification
    out_range_classes = zeros(1, numObjects);
    for i = 1:numObjects
        points3D = objectClouds{sortIdx(i)};
        u = (points3D(:,1) .* fx) ./ points3D(:,3) + cx;
        v = (points3D(:,2) .* fy) ./ points3D(:,3) + cy;
        uv = round([u, v]);
        
        validIndices = uv(:,1) >= 1 & uv(:,1) <= size(rgb,2) & ...
                       uv(:,2) >= 1 & uv(:,2) <= size(rgb,1);
        uvValid = uv(validIndices, :);
    
        mask = false(size(rgb,1), size(rgb,2));
        linearIndices = sub2ind(size(mask), uvValid(:,2), uvValid(:,1));
        mask(linearIndices) = true;
    
        xMin = max(min(uvValid(:,1)), 1);
        xMax = min(max(uvValid(:,1)), size(rgb,2));
        yMin = max(min(uvValid(:,2)), 1);
        yMax = min(max(uvValid(:,2)), size(rgb,1));
        bboxWidth = xMax - xMin + 1;
        bboxHeight = yMax - yMin + 1;
    
        maskedImg = rgb;
        bgColor = [11, 20, 43];
        for c = 1:3
            channel = maskedImg(:,:,c);
            channel(~mask) = bgColor(c);
            maskedImg(:,:,c) = channel;
        end
        
        cropped = imcrop(maskedImg, [xMin, yMin, bboxWidth-1, bboxHeight-1]);
        
        squareSize = max(bboxWidth, bboxHeight);
        squareImg = repmat(reshape(uint8(bgColor),1,1,3), squareSize, squareSize, 1);
        
        xOffset = floor((squareSize - bboxWidth)/2);
        yOffset = floor((squareSize - bboxHeight)/2);
        
        squareImg(yOffset+1:yOffset+bboxHeight,...
                 xOffset+1:xOffset+bboxWidth, :) = cropped;
        
        resized_size = [227 227];
        resizedImg = imresize(squareImg, resized_size, 'bilinear');  
        
        % run cnn
        class = classifier(resizedImg);
        out_range_classes(i) = class;

        rgb_filename = sprintf('Logs\\out_range_object%d_%d.png', int32(i), int32(class));
        imwrite(resizedImg, rgb_filename);
    end
end

function ypred  = classifier(image)
    isSim = coder.target('sfun');
    simSupported = false;
    useExtrinsic = isSim && ~simSupported;
    in_1 = single(image);
    [out_predict] = deep.blocks.internal.deepNetwork({in_1}, {size(in_1)}, {class(in_1)}, coder.const("SimulationSorting/To generate Config for robot"), 'classification_model.mat', useExtrinsic, true, 128, true, {'SSCB'}, {});
    [~, ypred] = max(out_predict);
end

function pose6D = hom2euler(T)
    x = T(1,4);
    y = T(2,4);
    z = T(3,4);
    
    R = T(1:3, 1:3);
    
    pitch = -asin(R(3,1));
    
    if abs(cos(pitch)) > 1e-5
        yaw = atan2(R(2,1)/cos(pitch), R(1,1)/cos(pitch));
        roll = atan2(R(3,2)/cos(pitch), R(3,3)/cos(pitch));
    else
        yaw = 0;
        roll = atan2(-R(1,2), R(2,2));
    end

    pose6D = [x, y, z, roll, pitch, yaw];
end

== matlab function SimulationSorting/Gripper Subsystem/MATLAB Function ==
  data: targetGrasped input; robotConfig output; gripperStatus input; inputConfig input; q_grip input
function robotConfig = appendGripper(targetGrasped, gripperStatus, inputConfig, q_grip)

persistent index
if isempty(index)
    index = 1;
end

% Open gripper
if ~gripperStatus
    openConfig = [0 0 0 0 0 0]';
    robotConfig = [inputConfig; openConfig]';
    index = 1;
else
    if index > size(q_grip, 2)
        robotConfig = [inputConfig; q_grip(:, index-1)]';
        index = 1;
    elseif targetGrasped
        robotConfig = [inputConfig; q_grip(:, index)]';
    else
        robotConfig = [inputConfig; q_grip(:, index)]';
        index = index + 1;
    end
end

== matlab function SimulationSorting/Camera Subsystem/MATLAB Function ==
  data: T input; Trans output; output output
function [Trans, output] = rotm2fixedZYX(T)
    R = T(1:3,1:3);
    Trans = T(1:3,4);
    if abs(R(3,1)) < 1
        pitch = -asin(R(3,1));
        roll  = atan2(R(3,2)/cos(pitch), R(3,3)/cos(pitch));
        yaw   = atan2(R(2,1)/cos(pitch), R(1,1)/cos(pitch));
    else
        % Gimbal lock
        if R(3,1) <= -1
            pitch = pi/2;
        else
            pitch = -pi/2;
        end
        yaw = 0;
        roll = atan2(-R(1,2), R(1,3));
    end
    output = [roll, pitch, yaw];
end
